simulink model "started"  (R2024b)
settings: Solver=VariableStepAuto  StartTime=0.0  StopTime=10.0  RelTol=1e-3
libraries: cstblocks x2
settings Model: Creator=manucoacci  LastModifiedBy=manucoacci

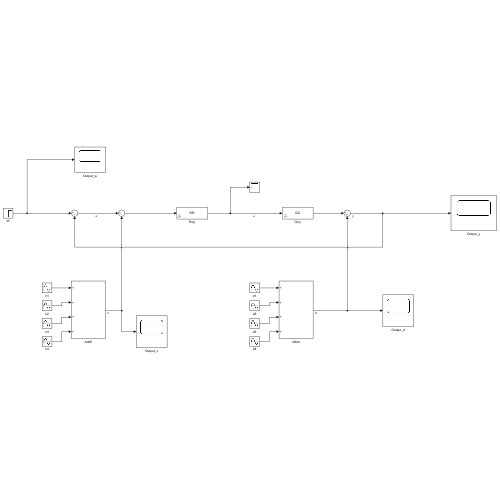
[thumbnail: Simulink's stored preview of the top-level diagram]
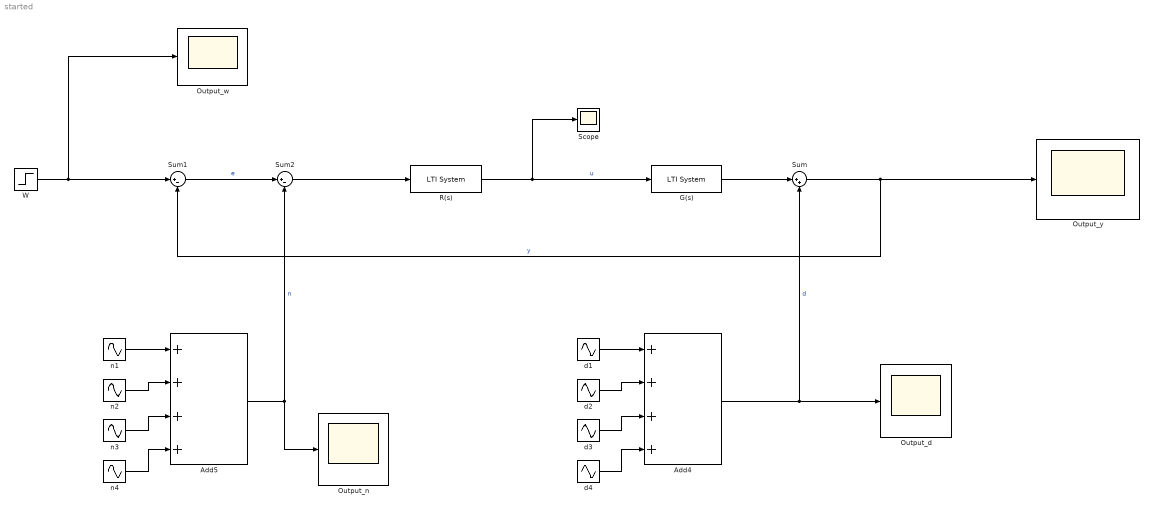
== system started ==
  Add4 : Sum  Inputs=++++
  Add5 : Sum  Inputs=++++
  G(s) : cstblocks/LTI System  sys=GG  IC=[]  PadeOrder=0
  Output_d : Scope
  Output_n : Scope
  Output_w : Scope
  Output_y : Scope
  R(s) : cstblocks/LTI System  sys=RR  IC=[]  PadeOrder=0
  Scope : Scope
  Sum : Sum  Inputs=|++
  Sum1 : Sum  Inputs=|+-
  Sum2 : Sum  Inputs=|+-
  W : Step  Time=0  After=2*pi()/3  SampleTime=0
  d1 : Sin  Amplitude=0.2  Frequency=0.1*1  SampleTime=0
  d2 : Sin  Amplitude=0.2  Frequency=0.1*2  SampleTime=0
  d3 : Sin  Amplitude=0.2  Frequency=0.1*3  SampleTime=0
  d4 : Sin  Amplitude=0.2  Frequency=0.1*4  SampleTime=0
  n1 : Sin  Amplitude=0.2  Frequency=10000*1  SampleTime=0
  n2 : Sin  Amplitude=0.2  Frequency=10000*2  SampleTime=0
  n3 : Sin  Amplitude=0.2  Frequency=10000*3  SampleTime=0
  n4 : Sin  Amplitude=0.2  Frequency=10000*4  SampleTime=0
  wires:
  Sum1/1 -> Sum2/1  "e"
  n2/1 -> Add5/2
  n1/1 -> Add5/1
  n4/1 -> Add5/4
  n3/1 -> Add5/3
  Add5/1 -> Output_n/1, Sum2/2  "n"
  Sum2/1 -> R(s)/1
  R(s)/1 -> Scope/1, G(s)/1  "u"
  G(s)/1 -> Sum/1
  d4/1 -> Add4/4
  d1/1 -> Add4/1
  d3/1 -> Add4/3
  d2/1 -> Add4/2
  Add4/1 -> Output_d/1, Sum/2  "d"
  Sum/1 -> Sum1/2, Output_y/1  "y"
  W/1 -> Output_w/1, Sum1/1
